simulink model "BoundedTorqueControl_2012b"  (Simulink 8.0)
settings: Solver=FixedStepDiscrete  StartTime=0.0  StopTime=CONFIG.SIMULATION_TIME  FixedStep=CONFIG.Ts  RelTol=1e-3
InitFcn:
  | cd(fileparts(which(bdroot)));
  | init_BoundedTorqueControl;
StopFcn:
  | visualization
values from neighbouring files (symbols this model uses):
  q0 = zeros(model.n, 1)    [gains.m]
  qd0 = zeros(model.n, 1)    [gains.m]
  ROBOT_DOF = model.n    [gains.m]
  ROBOT_DOF_SIM = eye(ROBOT_DOF)    [gains.m]
undefined symbols (not defined in the file or in its folder): CONFIG, DiscIntNeverNeededParam, model
settings Model: Creator=marie  LastModifiedBy=marie  CovModelRefEnable=off
settings DataIOCC: SaveFormat=StructureWithTime
settings OptimizationCC: ExpressionDepthLimit=128
settings DebuggingCC: UnderspecifiedInitializationDetection=Simplified  MergeDetectMultiDrivingBlocksExec=error  SolverPrmCheckMsg=none  FrameProcessingCompatibilityMsg=error  StateNameClashWarn=none
settings HardwareCC: ProdBitPerPointer=64  ProdLargestAtomicFloat=Float  ProdIntDivRoundTo=Zero  ProdEndianess=LittleEndian  ProdHWDeviceType=Specified
settings CodeAppCC: CustomSymbolStrType=$N$R$M_T
settings GRTTargetCC: CodeReplacementLibrary=C89/C90 (ANSI)  GeneratePreprocessorConditionals=Use local settings

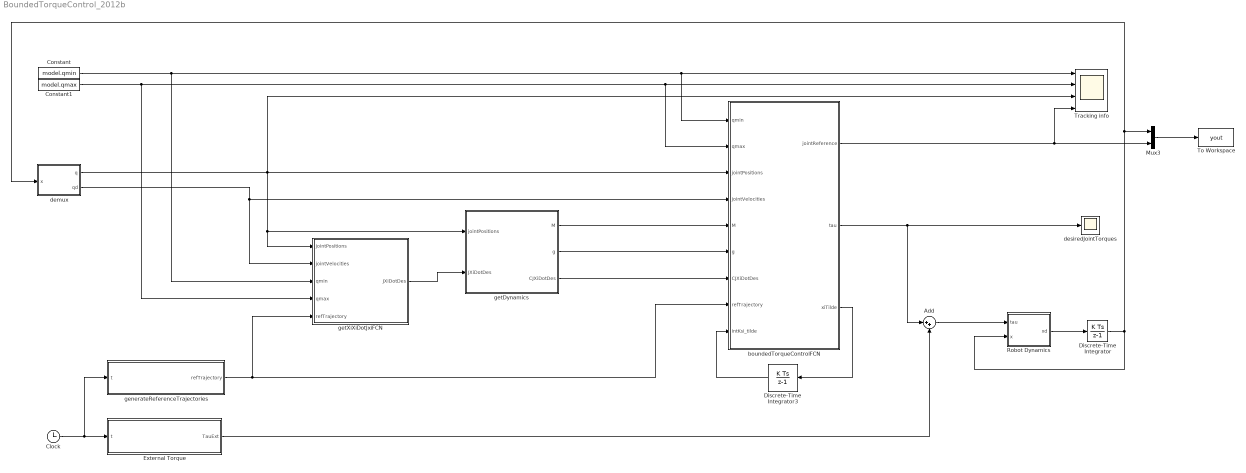
== system BoundedTorqueControl_2012b ==
  Add : Sum  Inputs=|++
  Clock : Clock
  Constant : Constant  Value=model.qmin
  Constant1 : Constant  Value=model.qmax
  Discrete-Time Integrator : DiscreteIntegrator  InitialCondition=[q0; qd0]  InitialConditionMode=State only (most efficient)  SampleTime=CONFIG.Ts  ICPrevOutput=DiscIntNeverNeededParam  ICPrevScaledInput=DiscIntNeverNeededParam
  Discrete-Time Integrator3 : DiscreteIntegrator  InitialCondition=zeros(ROBOT_DOF,1)  InitialConditionMode=State only (most efficient)  SampleTime=CONFIG.Ts  ICPrevOutput=DiscIntNeverNeededParam  ICPrevScaledInput=DiscIntNeverNeededParam
  External Torque : MATLAB Function  TreatAsAtomicUnit=on
      settings: PermitHierarchicalResolution=ParametersOnly
  Mux3 : Mux  Inputs=2
  Robot Dynamics : MATLAB Function  TreatAsAtomicUnit=on
      settings: PermitHierarchicalResolution=ParametersOnly
  To Workspace : ToWorkspace  VariableName=yout  SaveFormat=Structure With Time  SampleTime=-1
  Tracking info : Scope  NumInputPorts=4
      settings: TimeRange=auto  MaxDataPoints=5000  SaveToWorkspace=off  SaveName=ScopeData3  YMin=-3.92699~-5~-5~-5  YMax=3.92699~5~5~5  SampleTime=-1
  boundedTorqueControlFCN : MATLAB Function  TreatAsAtomicUnit=on
      settings: PermitHierarchicalResolution=ParametersOnly
  demux : MATLAB Function  TreatAsAtomicUnit=on
      settings: PermitHierarchicalResolution=ParametersOnly
  desiredJointTorques : Scope
      settings: TimeRange=auto  MaxDataPoints=5000  SaveToWorkspace=off  SaveName=ScopeData2  YMin=-37.89261  YMax=80.85971  SampleTime=-1
  generateReferenceTrajectories : MATLAB Function  TreatAsAtomicUnit=on
      settings: PermitHierarchicalResolution=ParametersOnly
  getDynamics : MATLAB Function  TreatAsAtomicUnit=on
      settings: PermitHierarchicalResolution=ParametersOnly
  getXiXiDotJxiFCN : MATLAB Function  TreatAsAtomicUnit=on
      settings: PermitHierarchicalResolution=ParametersOnly
  wires:
  demux/1(q) -> getDynamics/1(jointPositions), getXiXiDotJxiFCN/1(jointPositions), boundedTorqueControlFCN/3(jointPositions), Tracking info/3
  demux/2(qd) -> boundedTorqueControlFCN/4(jointVelocities), getXiXiDotJxiFCN/2(jointVelocities)
  getDynamics/1(M) -> boundedTorqueControlFCN/5(M)
  Constant1/1 -> getXiXiDotJxiFCN/4(qmax), boundedTorqueControlFCN/2(qmax), Tracking info/2
  Constant/1 -> boundedTorqueControlFCN/1(qmin), Tracking info/1, getXiXiDotJxiFCN/3(qmin)
  boundedTorqueControlFCN/2(tau) -> Add/1, desiredJointTorques/1
  Discrete-Time Integrator3/1 -> boundedTorqueControlFCN/9(intKsi_tilde)
  Clock/1 -> generateReferenceTrajectories/1(t), External Torque/1(t)
  External Torque/1(TauExt) -> Add/2
  boundedTorqueControlFCN/1(jointReference) -> Tracking info/4, Mux3/2
  getDynamics/2(g) -> boundedTorqueControlFCN/6(g)
  getXiXiDotJxiFCN/1(JXiDotDes) -> getDynamics/2(JXiDotDes)
  getDynamics/3(CJXiDotDes) -> boundedTorqueControlFCN/7(CJXiDotDes)
  boundedTorqueControlFCN/3(xiTilde) -> Discrete-Time Integrator3/1
  Add/1 -> Robot Dynamics/1(tau)
  Robot Dynamics/1(xd) -> Discrete-Time Integrator/1
  Discrete-Time Integrator/1 -> demux/1(x), Mux3/1, Robot Dynamics/2(x)
  Mux3/1 -> To Workspace/1
  generateReferenceTrajectories/1(refTrajectory) -> getXiXiDotJxiFCN/5(refTrajectory), boundedTorqueControlFCN/8(refTrajectory)

== matlab function boundedTorqueControlFCN ==
  data: model parameter double; qmin input double; qmax input double; jointReference output double; jointPositions input double; jointVelocities input double; M input double; g input double; CJXiDotDes input double; refTrajectory input double; intKsi_tilde input double; tau output double; xiTilde output double
function [jointReference, tau, xiTilde] =  boundedJointEvolutionControl(model, qmin, qmax, jointPositions, jointVelocities, M, g, CJXiDotDes, refTrajectory, intKsi_tilde)


    [~, ~, jointReference, ~, tau, xiTilde] = boundedJointEvolutionControl(model, qmin, qmax, jointPositions, jointVelocities, M, g, CJXiDotDes, refTrajectory, intKsi_tilde);

== matlab function generateReferenceTrajectories ==
  data: refTrajectory output double; t input double; model parameter double; ROBOT_DOF_SIM parameter double
function refTrajectory  = generateReferenceTrajectoriesFCN(t, model,ROBOT_DOF_SIM)

% refTrajectory  = ones(size(ROBOT_DOF_SIM,1),1)*generateReferenceTrajectories(t, model);

refTrajectory  = generateReferenceTrajectories(t, model);

== matlab function External Torque ==
  data: TauExt output double; t input double; model parameter double
function TauExt = applyExternTorqueFCN(t, model)

TauExt = applyExternTorque(t, model);

== matlab function getXiXiDotJxiFCN ==
  data: JXiDotDes output double; jointPositions input double; jointVelocities input double; qmin input double; qmax input double; refTrajectory input double
function JXiDotDes  = getXiXiDotJxiFCN(jointPositions,jointVelocities, qmin, qmax, refTrajectory)


[~,~,J,~]        = getXiXiDotJxi(jointPositions,jointVelocities,qmin, qmax);

[r,rDot,~]       = getReferences(refTrajectory);

[~,xiDotDes,~,~] = getXiXiDotJxi(r,rDot,qmin, qmax);

JXiDotDes        = J*xiDotDes;

== matlab function Robot Dynamics ==
  data: tau input double; x input double; xd output double; model parameter double
function xd = getDyn(tau, x, model)

%Compute the dynamics of the system, 
%from the parameters in model
%following Siciliano, p.268

%Input:
%Tau: control torques
%x = [q; qd] = [x1; x2]
%model: model parameters set in init script

%Output:
%xd = [qd; qdd] = [x2; M\(tau - h(q,qd))]

q = x(1:2);
qd = x(3:4);

Fv = model.Fv;

%M matrix
M = computeMSiciliano(q,model);

%C matrix
C = computeCSiciliano(q,qd,model);

%G matrix
G = computeGSiciliano(q, model);


qdd = M \ (tau - C*qd - Fv*qd - G);

xd = [qd; qdd];

end

== matlab function getDynamics ==
  data: jointPositions input double; JXiDotDes input double; M output double; g output double; CJXiDotDes output double; model parameter double
function [M, g, CJXiDotDes] = getDynamics(jointPositions, JXiDotDes, model)


M = computeMSiciliano(jointPositions, model);

g = computeGSiciliano(jointPositions, model);

CJXiDotDes = computeCSiciliano(jointPositions, JXiDotDes, model) * JXiDotDes;

== matlab function demux ==
  data: x input double; q output double; qd output double
function [q, qd] = getq(x)

%From the dynamics output x, extract the joint positions and velocities

%Input
%x: state of the system in the form [q;qd], output from the dynamic model

%Output
%q: joint positions
%qd: joint velocities

q = x(1:2);
q(1) = q(1);
qd = x(3:4);
